simulink model "pfb_fir_256c_2p_16i_8b_core"  (R2019a)
(part 3 of 29)

      mask prompts: mult_latency "Multiplier Latency"; coeff_width "Coefficient Bit Width In"; coeff_frac_width "Coefficient Fractional Bits"; delay "Data/Sync Delay"; data_width "Data Bit Width In"; bram_latency "BRAM Latency"; use_hdl "Use behavioral HDL for multlipliers"; use_embedded "Use embedded multipliers"
      mask init: same as pfb_fir_256c_2p_16i_8b_core/pfb_fir/pol1_in10_tap2
      mask Callback use_hdl:
      | use_hdl = get_param(gcb,'use_hdl');
      | if( strcmp(use_hdl,'on')),
      |     set_param(gcb, 'use_embedded','off');
      |     set_param(gcb, 'MaskVisibilities',{'on','on','on','on','on','on','on','off'});
      | else,
      |     set_param(gcb, 'MaskVisibilities',{'on','on','on','on','on','on','on','on'});
      | end
  pol1_in8_tap7 : Subsystem  AncestorBlock=casper_library_pfbs/tap  mask(tap){mult_latency=2, coeff_width=18, coeff_frac_width=17, delay=16, data_width=8, bram_latency=2, use_hdl=on, use_embedded=off}
      mask prompts: mult_latency "Multiplier Latency"; coeff_width "Coefficient Bit Width In"; coeff_frac_width "Coefficient Fractional Bits"; delay "Data/Sync Delay"; data_width "Data Bit Width In"; bram_latency "BRAM Latency"; use_hdl "Use behavioral HDL for multlipliers"; use_embedded "Use embedded multipliers"
      mask init: same as pfb_fir_256c_2p_16i_8b_core/pfb_fir/pol1_in10_tap2
      mask Callback use_hdl:
      | use_hdl = get_param(gcb,'use_hdl');
      | if( strcmp(use_hdl,'on')),
      |     set_param(gcb, 'use_embedded','off');
      |     set_param(gcb, 'MaskVisibilities',{'on','on','on','on','on','on','on','off'});
      | else,
      |     set_param(gcb, 'MaskVisibilities',{'on','on','on','on','on','on','on','on'});
      | end
  pol1_in9_coeffs : Subsystem  AncestorBlock=casper_library_pfbs/pfb_coeff_gen  mask(pfb_coeff_gen){PFBSize=8, CoeffBitWidth=18, TotalTaps=8, CoeffDistMem=off, WindowType=hamming, bram_latency=2, n_inputs=4, nput=8, fwidth=1, debug_mode=off, fan_latency=1}
      mask prompts: PFBSize "Size of PFB: (2^? pnts)"; CoeffBitWidth "Bitwidth of Coefficients:"; TotalTaps "Total Number of Taps:"; CoeffDistMem "Implement Coeff Gen in Distributed Memory"; WindowType "Windowing Function:"; bram_latency "BRAM Latency"; n_inputs "Number of Simultaneous Inputs: (2^?)"; nput "This is input number:"; fwidth "Bin Width (normal=1)"; debug_mode "Debug mode - coeffs are a [1:pfb_size*taps] ramp."; fan_latency "Fanout latency"
      mask init: same as pfb_fir_256c_2p_16i_8b_core/pfb_fir/pol1_in10_coeffs
      settings: AttributesFormatString=|
      | PFBSize=8, n_inputs=4,
      | taps=8, input=8
  pol1_in9_first_tap : Subsystem  AncestorBlock=casper_library_pfbs/first_tap  mask(first_tap){PFBSize=8, CoeffBitWidth=18, TotalTaps=8, BitWidthIn=8, WindowType=hamming, mult_latency=2, bram_latency=2, n_inputs=4, fwidth=1, use_hdl=on, use_embedded=off}
      mask prompts: PFBSize "Size of PFB: (2^? pnts)"; CoeffBitWidth "Bitwidth of Coefficients:"; TotalTaps "Total Number of Taps:"; BitWidthIn "Input Bitwidth:"; WindowType "Windowing Function:"; mult_latency "Mult Latency"; bram_latency "BRAM Latency"; n_inputs "Number of Simultaneous Inputs: (2^?)"; fwidth "Bit Width (normal=1)"; use_hdl "Use behavioral HDL for multlipliers"; use_embedded "Use embedded multipliers"
      mask init: same as pfb_fir_256c_2p_16i_8b_core/pfb_fir/pol1_in10_first_tap
      settings: AttributesFormatString=taps=8
      mask TypeOptions WindowType: bartlett | barthannwin | blackman | blackmanharris | bohamwin | chebwin | flattopwin | gausswin | hamming | hann | kaiser | nuttallwin | parzenwin | rectwin | tukeywin | triang
      mask Callback use_hdl:
      | use_hdl = get_param(gcb,'use_hdl');
      | if( strcmp(use_hdl,'on')),
      |     set_param(gcb, 'use_embedded','off');
      |     set_param(gcb, 'MaskVisibilities',{'on','on','on','on','on','on','on','on','on','on','off'});
      | else,
      |     set_param(gcb, 'MaskVisibilities',{'on','on','on','on','on','on','on','on','on','on','on'});
      | end
  pol1_in9_last_tap : Subsystem  AncestorBlock=casper_library_pfbs/last_tap  mask(last_tap){TotalTaps=8, BitWidthIn=8, BitWidthOut=18, CoeffBitWidth=18, add_latency=1, mult_latency=2, quantization=Round  (unbiased: Even Values), use_hdl=on, use_embedded=off}
      mask prompts: TotalTaps "Total Number of Taps:"; BitWidthIn "Input Bitwidth:"; BitWidthOut "Output Bitwidth:"; CoeffBitWidth "Coeff Bitwidth:"; add_latency "Add Latency"; mult_latency "Mult Latency"; quantization "Quantization Behavior"; use_hdl "Use behavioral HDL for multlipliers"; use_embedded "Use embedded multipliers"
      mask init: same as pfb_fir_256c_2p_16i_8b_core/pfb_fir/pol1_in10_last_tap
      settings: AttributesFormatString=taps=8
      mask TypeOptions quantization: Truncate | Round  (unbiased: +/- Inf) | Round  (unbiased: Even Values)
      mask Callback use_hdl:
      | use_hdl = get_param(gcb,'use_hdl');
      | if( strcmp(use_hdl,'on')),
      |     set_param(gcb, 'use_embedded','off');
      |     set_param(gcb, 'MaskVisibilities',{'on','on','on','on','on','on','on','on','off'});
      | else,
      |     set_param(gcb, 'MaskVisibilities',{'on','on','on','on','on','on','on','on','on'});
      | end
  pol1_in9_tap2 : Subsystem  AncestorBlock=casper_library_pfbs/tap  mask(tap){mult_latency=2, coeff_width=18, coeff_frac_width=17, delay=16, data_width=8, bram_latency=2, use_hdl=on, use_embedded=off}
      mask prompts: mult_latency "Multiplier Latency"; coeff_width "Coefficient Bit Width In"; coeff_frac_width "Coefficient Fractional Bits"; delay "Data/Sync Delay"; data_width "Data Bit Width In"; bram_latency "BRAM Latency"; use_hdl "Use behavioral HDL for multlipliers"; use_embedded "Use embedded multipliers"
      mask init: same as pfb_fir_256c_2p_16i_8b_core/pfb_fir/pol1_in10_tap2
      mask Callback use_hdl:
      | use_hdl = get_param(gcb,'use_hdl');
      | if( strcmp(use_hdl,'on')),
      |     set_param(gcb, 'use_embedded','off');
      |     set_param(gcb, 'MaskVisibilities',{'on','on','on','on','on','on','on','off'});
      | else,
      |     set_param(gcb, 'MaskVisibilities',{'on','on','on','on','on','on','on','on'});
      | end
  pol1_in9_tap3 : Subsystem  AncestorBlock=casper_library_pfbs/tap  mask(tap){mult_latency=2, coeff_width=18, coeff_frac_width=17, delay=16, data_width=8, bram_latency=2, use_hdl=on, use_embedded=off}
      mask prompts: mult_latency "Multiplier Latency"; coeff_width "Coefficient Bit Width In"; coeff_frac_width "Coefficient Fractional Bits"; delay "Data/Sync Delay"; data_width "Data Bit Width In"; bram_latency "BRAM Latency"; use_hdl "Use behavioral HDL for multlipliers"; use_embedded "Use embedded multipliers"
      mask init: same as pfb_fir_256c_2p_16i_8b_core/pfb_fir/pol1_in10_tap2
      mask Callback use_hdl:
      | use_hdl = get_param(gcb,'use_hdl');
      | if( strcmp(use_hdl,'on')),
      |     set_param(gcb, 'use_embedded','off');
      |     set_param(gcb, 'MaskVisibilities',{'on','on','on','on','on','on','on','off'});
      | else,
      |     set_param(gcb, 'MaskVisibilities',{'on','on','on','on','on','on','on','on'});
      | end
  pol1_in9_tap4 : Subsystem  AncestorBlock=casper_library_pfbs/tap  mask(tap){mult_latency=2, coeff_width=18, coeff_frac_width=17, delay=16, data_width=8, bram_latency=2, use_hdl=on, use_embedded=off}
      mask prompts: mult_latency "Multiplier Latency"; coeff_width "Coefficient Bit Width In"; coeff_frac_width "Coefficient Fractional Bits"; delay "Data/Sync Delay"; data_width "Data Bit Width In"; bram_latency "BRAM Latency"; use_hdl "Use behavioral HDL for multlipliers"; use_embedded "Use embedded multipliers"
      mask init: same as pfb_fir_256c_2p_16i_8b_core/pfb_fir/pol1_in10_tap2
      mask Callback use_hdl:
      | use_hdl = get_param(gcb,'use_hdl');
      | if( strcmp(use_hdl,'on')),
      |     set_param(gcb, 'use_embedded','off');
      |     set_param(gcb, 'MaskVisibilities',{'on','on','on','on','on','on','on','off'});
      | else,
      |     set_param(gcb, 'MaskVisibilities',{'on','on','on','on','on','on','on','on'});
      | end
  pol1_in9_tap5 : Subsystem  AncestorBlock=casper_library_pfbs/tap  mask(tap){mult_latency=2, coeff_width=18, coeff_frac_width=17, delay=16, data_width=8, bram_latency=2, use_hdl=on, use_embedded=off}
      mask prompts: mult_latency "Multiplier Latency"; coeff_width "Coefficient Bit Width In"; coeff_frac_width "Coefficient Fractional Bits"; delay "Data/Sync Delay"; data_width "Data Bit Width In"; bram_latency "BRAM Latency"; use_hdl "Use behavioral HDL for multlipliers"; use_embedded "Use embedded multipliers"
      mask init: same as pfb_fir_256c_2p_16i_8b_core/pfb_fir/pol1_in10_tap2
      mask Callback use_hdl:
      | use_hdl = get_param(gcb,'use_hdl');
      | if( strcmp(use_hdl,'on')),
      |     set_param(gcb, 'use_embedded','off');
      |     set_param(gcb, 'MaskVisibilities',{'on','on','on','on','on','on','on','off'});
      | else,
      |     set_param(gcb, 'MaskVisibilities',{'on','on','on','on','on','on','on','on'});
      | end
  pol1_in9_tap6 : Subsystem  AncestorBlock=casper_library_pfbs/tap  mask(tap){mult_latency=2, coeff_width=18, coeff_frac_width=17, delay=16, data_width=8, bram_latency=2, use_hdl=on, use_embedded=off}
      mask prompts: mult_latency "Multiplier Latency"; coeff_width "Coefficient Bit Width In"; coeff_frac_width "Coefficient Fractional Bits"; delay "Data/Sync Delay"; data_width "Data Bit Width In"; bram_latency "BRAM Latency"; use_hdl "Use behavioral HDL for multlipliers"; use_embedded "Use embedded multipliers"
      mask init: same as pfb_fir_256c_2p_16i_8b_core/pfb_fir/pol1_in10_tap2
      mask Callback use_hdl:
      | use_hdl = get_param(gcb,'use_hdl');
      | if( strcmp(use_hdl,'on')),
      |     set_param(gcb, 'use_embedded','off');
      |     set_param(gcb, 'MaskVisibilities',{'on','on','on','on','on','on','on','off'});
      | else,
      |     set_param(gcb, 'MaskVisibilities',{'on','on','on','on','on','on','on','on'});
      | end
  pol1_in9_tap7 : Subsystem  AncestorBlock=casper_library_pfbs/tap  mask(tap){mult_latency=2, coeff_width=18, coeff_frac_width=17, delay=16, data_width=8, bram_latency=2, use_hdl=on, use_embedded=off}
      mask prompts: mult_latency "Multiplier Latency"; coeff_width "Coefficient Bit Width In"; coeff_frac_width "Coefficient Fractional Bits"; delay "Data/Sync Delay"; data_width "Data Bit Width In"; bram_latency "BRAM Latency"; use_hdl "Use behavioral HDL for multlipliers"; use_embedded "Use embedded multipliers"
      mask init: same as pfb_fir_256c_2p_16i_8b_core/pfb_fir/pol1_in10_tap2
      mask Callback use_hdl:
      | use_hdl = get_param(gcb,'use_hdl');
      | if( strcmp(use_hdl,'on')),
      |     set_param(gcb, 'use_embedded','off');
      |     set_param(gcb, 'MaskVisibilities',{'on','on','on','on','on','on','on','off'});
      | else,
      |     set_param(gcb, 'MaskVisibilities',{'on','on','on','on','on','on','on','on'});
      | end
  sync_out : Outport
  pol1_out1 : Outport  Port=2
  pol1_out2 : Outport  Port=3
  pol1_out3 : Outport  Port=4
  pol1_out4 : Outport  Port=5
  pol1_out5 : Outport  Port=6
  pol1_out6 : Outport  Port=7
  pol1_out7 : Outport  Port=8
  pol1_out8 : Outport  Port=9
  pol1_out9 : Outport  Port=10
  pol1_out10 : Outport  Port=11
  pol1_out11 : Outport  Port=12
  pol1_out12 : Outport  Port=13
  pol1_out13 : Outport  Port=14
  pol1_out14 : Outport  Port=15
  pol1_out15 : Outport  Port=16
  pol1_out16 : Outport  Port=17
  wires:
  pol1_in1/1 -> pol1_in1_coeffs/1(din)
  sync/1 -> pol1_in1_coeffs/2(sync), pol1_in2_coeffs/2(sync), pol1_in3_coeffs/2(sync), pol1_in4_coeffs/2(sync), pol1_in5_coeffs/2(sync), pol1_in6_coeffs/2(sync), pol1_in7_coeffs/2(sync), pol1_in8_coeffs/2(sync), pol1_in9_coeffs/2(sync), pol1_in10_coeffs/2(sync), pol1_in11_coeffs/2(sync), pol1_in12_coeffs/2(sync), pol1_in13_coeffs/2(sync), pol1_in14_coeffs/2(sync), pol1_in15_coeffs/2(sync), pol1_in16_coeffs/2(sync)
  pol1_in1_coeffs/1(dout) -> pol1_in1_first_tap/1(din)
  pol1_in1_coeffs/2(sync_out) -> pol1_in1_first_tap/2(sync), pol1_in2_first_tap/2(sync), pol1_in3_first_tap/2(sync), pol1_in4_first_tap/2(sync), pol1_in5_first_tap/2(sync), pol1_in6_first_tap/2(sync), pol1_in7_first_tap/2(sync), pol1_in8_first_tap/2(sync), pol1_in9_first_tap/2(sync), pol1_in10_first_tap/2(sync), pol1_in11_first_tap/2(sync), pol1_in12_first_tap/2(sync), pol1_in13_first_tap/2(sync), pol1_in14_first_tap/2(sync), pol1_in15_first_tap/2(sync), pol1_in16_first_tap/2(sync)
  pol1_in1_coeffs/3(coeff) -> pol1_in1_first_tap/3(coeffs)
  pol1_in1_first_tap/1(dout) -> pol1_in1_tap2/1(din)
  pol1_in1_first_tap/2(sync_out) -> pol1_in1_tap2/2(sync)
  pol1_in1_first_tap/3(coeff_out) -> pol1_in1_tap2/3(coeff)
  pol1_in1_first_tap/4(taps_out) -> pol1_in1_tap2/4(taps)
  pol1_in1_tap2/1(dout) -> pol1_in1_tap3/1(din)
  pol1_in1_tap2/2(sync_out) -> pol1_in1_tap3/2(sync)
  pol1_in1_tap2/3(coeff_out) -> pol1_in1_tap3/3(coeff)
  pol1_in1_tap2/4(taps_out) -> pol1_in1_tap3/4(taps)
  pol1_in1_tap3/1(dout) -> pol1_in1_tap4/1(din)
  pol1_in1_tap3/2(sync_out) -> pol1_in1_tap4/2(sync)
  pol1_in1_tap3/3(coeff_out) -> pol1_in1_tap4/3(coeff)
  pol1_in1_tap3/4(taps_out) -> pol1_in1_tap4/4(taps)
  pol1_in1_tap4/1(dout) -> pol1_in1_tap5/1(din)
  pol1_in1_tap4/2(sync_out) -> pol1_in1_tap5/2(sync)
  pol1_in1_tap4/3(coeff_out) -> pol1_in1_tap5/3(coeff)
  pol1_in1_tap4/4(taps_out) -> pol1_in1_tap5/4(taps)
  pol1_in1_tap5/1(dout) -> pol1_in1_tap6/1(din)
  pol1_in1_tap5/2(sync_out) -> pol1_in1_tap6/2(sync)
  pol1_in1_tap5/3(coeff_out) -> pol1_in1_tap6/3(coeff)
  pol1_in1_tap5/4(taps_out) -> pol1_in1_tap6/4(taps)
  pol1_in1_tap6/1(dout) -> pol1_in1_tap7/1(din)
  pol1_in1_tap6/2(sync_out) -> pol1_in1_tap7/2(sync)
  pol1_in1_tap6/3(coeff_out) -> pol1_in1_tap7/3(coeff)
  pol1_in1_tap6/4(taps_out) -> pol1_in1_tap7/4(taps)
  pol1_in1_tap7/1(dout) -> pol1_in1_last_tap/1(din)
  pol1_in1_tap7/2(sync_out) -> pol1_in1_last_tap/2(sync)
  pol1_in1_tap7/3(coeff_out) -> pol1_in1_last_tap/3(coeff)
  pol1_in1_tap7/4(taps_out) -> pol1_in1_last_tap/4(taps)
  pol1_in1_last_tap/1(dout) -> pol1_out1/1
  pol1_in1_last_tap/2(sync_out) -> sync_out/1
  pol1_in2/1 -> pol1_in2_coeffs/1(din)
  pol1_in2_coeffs/1(dout) -> pol1_in2_first_tap/1(din)
  pol1_in2_coeffs/3(coeff) -> pol1_in2_first_tap/3(coeffs)
  pol1_in2_first_tap/1(dout) -> pol1_in2_tap2/1(din)
  pol1_in2_first_tap/2(sync_out) -> pol1_in2_tap2/2(sync)
  pol1_in2_first_tap/3(coeff_out) -> pol1_in2_tap2/3(coeff)
  pol1_in2_first_tap/4(taps_out) -> pol1_in2_tap2/4(taps)
  pol1_in2_tap2/1(dout) -> pol1_in2_tap3/1(din)
  pol1_in2_tap2/2(sync_out) -> pol1_in2_tap3/2(sync)
  pol1_in2_tap2/3(coeff_out) -> pol1_in2_tap3/3(coeff)
  pol1_in2_tap2/4(taps_out) -> pol1_in2_tap3/4(taps)
  pol1_in2_tap3/1(dout) -> pol1_in2_tap4/1(din)
  pol1_in2_tap3/2(sync_out) -> pol1_in2_tap4/2(sync)
  pol1_in2_tap3/3(coeff_out) -> pol1_in2_tap4/3(coeff)
  pol1_in2_tap3/4(taps_out) -> pol1_in2_tap4/4(taps)
  pol1_in2_tap4/1(dout) -> pol1_in2_tap5/1(din)
  pol1_in2_tap4/2(sync_out) -> pol1_in2_tap5/2(sync)
  pol1_in2_tap4/3(coeff_out) -> pol1_in2_tap5/3(coeff)
  pol1_in2_tap4/4(taps_out) -> pol1_in2_tap5/4(taps)
  pol1_in2_tap5/1(dout) -> pol1_in2_tap6/1(din)
  pol1_in2_tap5/2(sync_out) -> pol1_in2_tap6/2(sync)
  pol1_in2_tap5/3(coeff_out) -> pol1_in2_tap6/3(coeff)
  pol1_in2_tap5/4(taps_out) -> pol1_in2_tap6/4(taps)
  pol1_in2_tap6/1(dout) -> pol1_in2_tap7/1(din)
  pol1_in2_tap6/2(sync_out) -> pol1_in2_tap7/2(sync)
  pol1_in2_tap6/3(coeff_out) -> pol1_in2_tap7/3(coeff)
  pol1_in2_tap6/4(taps_out) -> pol1_in2_tap7/4(taps)
  pol1_in2_tap7/1(dout) -> pol1_in2_last_tap/1(din)
  pol1_in2_tap7/2(sync_out) -> pol1_in2_last_tap/2(sync)
  pol1_in2_tap7/3(coeff_out) -> pol1_in2_last_tap/3(coeff)
  pol1_in2_tap7/4(taps_out) -> pol1_in2_last_tap/4(taps)
  pol1_in2_last_tap/1(dout) -> pol1_out2/1
  pol1_in3/1 -> pol1_in3_coeffs/1(din)
  pol1_in3_coeffs/1(dout) -> pol1_in3_first_tap/1(din)
  pol1_in3_coeffs/3(coeff) -> pol1_in3_first_tap/3(coeffs)
  pol1_in3_first_tap/1(dout) -> pol1_in3_tap2/1(din)
  pol1_in3_first_tap/2(sync_out) -> pol1_in3_tap2/2(sync)
  pol1_in3_first_tap/3(coeff_out) -> pol1_in3_tap2/3(coeff)
  pol1_in3_first_tap/4(taps_out) -> pol1_in3_tap2/4(taps)
  pol1_in3_tap2/1(dout) -> pol1_in3_tap3/1(din)
  pol1_in3_tap2/2(sync_out) -> pol1_in3_tap3/2(sync)
  pol1_in3_tap2/3(coeff_out) -> pol1_in3_tap3/3(coeff)
  pol1_in3_tap2/4(taps_out) -> pol1_in3_tap3/4(taps)
  pol1_in3_tap3/1(dout) -> pol1_in3_tap4/1(din)
  pol1_in3_tap3/2(sync_out) -> pol1_in3_tap4/2(sync)
  pol1_in3_tap3/3(coeff_out) -> pol1_in3_tap4/3(coeff)
  pol1_in3_tap3/4(taps_out) -> pol1_in3_tap4/4(taps)
  pol1_in3_tap4/1(dout) -> pol1_in3_tap5/1(din)
  pol1_in3_tap4/2(sync_out) -> pol1_in3_tap5/2(sync)
  pol1_in3_tap4/3(coeff_out) -> pol1_in3_tap5/3(coeff)
  pol1_in3_tap4/4(taps_out) -> pol1_in3_tap5/4(taps)
  pol1_in3_tap5/1(dout) -> pol1_in3_tap6/1(din)
  pol1_in3_tap5/2(sync_out) -> pol1_in3_tap6/2(sync)
  pol1_in3_tap5/3(coeff_out) -> pol1_in3_tap6/3(coeff)
  pol1_in3_tap5/4(taps_out) -> pol1_in3_tap6/4(taps)
  pol1_in3_tap6/1(dout) -> pol1_in3_tap7/1(din)
  pol1_in3_tap6/2(sync_out) -> pol1_in3_tap7/2(sync)
  pol1_in3_tap6/3(coeff_out) -> pol1_in3_tap7/3(coeff)
  pol1_in3_tap6/4(taps_out) -> pol1_in3_tap7/4(taps)
  pol1_in3_tap7/1(dout) -> pol1_in3_last_tap/1(din)
  pol1_in3_tap7/2(sync_out) -> pol1_in3_last_tap/2(sync)
  pol1_in3_tap7/3(coeff_out) -> pol1_in3_last_tap/3(coeff)
  pol1_in3_tap7/4(taps_out) -> pol1_in3_last_tap/4(taps)
  pol1_in3_last_tap/1(dout) -> pol1_out3/1
  pol1_in4/1 -> pol1_in4_coeffs/1(din)
  pol1_in4_coeffs/1(dout) -> pol1_in4_first_tap/1(din)
  pol1_in4_coeffs/3(coeff) -> pol1_in4_first_tap/3(coeffs)
  pol1_in4_first_tap/1(dout) -> pol1_in4_tap2/1(din)
  pol1_in4_first_tap/2(sync_out) -> pol1_in4_tap2/2(sync)
  pol1_in4_first_tap/3(coeff_out) -> pol1_in4_tap2/3(coeff)
  pol1_in4_first_tap/4(taps_out) -> pol1_in4_tap2/4(taps)
  pol1_in4_tap2/1(dout) -> pol1_in4_tap3/1(din)
  pol1_in4_tap2/2(sync_out) -> pol1_in4_tap3/2(sync)
  pol1_in4_tap2/3(coeff_out) -> pol1_in4_tap3/3(coeff)
  pol1_in4_tap2/4(taps_out) -> pol1_in4_tap3/4(taps)
  pol1_in4_tap3/1(dout) -> pol1_in4_tap4/1(din)
  pol1_in4_tap3/2(sync_out) -> pol1_in4_tap4/2(sync)
  pol1_in4_tap3/3(coeff_out) -> pol1_in4_tap4/3(coeff)
  pol1_in4_tap3/4(taps_out) -> pol1_in4_tap4/4(taps)
  pol1_in4_tap4/1(dout) -> pol1_in4_tap5/1(din)
  pol1_in4_tap4/2(sync_out) -> pol1_in4_tap5/2(sync)
  pol1_in4_tap4/3(coeff_out) -> pol1_in4_tap5/3(coeff)
  pol1_in4_tap4/4(taps_out) -> pol1_in4_tap5/4(taps)
  pol1_in4_tap5/1(dout) -> pol1_in4_tap6/1(din)
  pol1_in4_tap5/2(sync_out) -> pol1_in4_tap6/2(sync)
  pol1_in4_tap5/3(coeff_out) -> pol1_in4_tap6/3(coeff)
  pol1_in4_tap5/4(taps_out) -> pol1_in4_tap6/4(taps)
  pol1_in4_tap6/1(dout) -> pol1_in4_tap7/1(din)
  pol1_in4_tap6/2(sync_out) -> pol1_in4_tap7/2(sync)
  pol1_in4_tap6/3(coeff_out) -> pol1_in4_tap7/3(coeff)
  pol1_in4_tap6/4(taps_out) -> pol1_in4_tap7/4(taps)
  pol1_in4_tap7/1(dout) -> pol1_in4_last_tap/1(din)
  pol1_in4_tap7/2(sync_out) -> pol1_in4_last_tap/2(sync)
  pol1_in4_tap7/3(coeff_out) -> pol1_in4_last_tap/3(coeff)
  pol1_in4_tap7/4(taps_out) -> pol1_in4_last_tap/4(taps)
  pol1_in4_last_tap/1(dout) -> pol1_out4/1
  pol1_in5/1 -> pol1_in5_coeffs/1(din)
  pol1_in5_coeffs/1(dout) -> pol1_in5_first_tap/1(din)
  pol1_in5_coeffs/3(coeff) -> pol1_in5_first_tap/3(coeffs)
  pol1_in5_first_tap/1(dout) -> pol1_in5_tap2/1(din)
  pol1_in5_first_tap/2(sync_out) -> pol1_in5_tap2/2(sync)
  pol1_in5_first_tap/3(coeff_out) -> pol1_in5_tap2/3(coeff)
  pol1_in5_first_tap/4(taps_out) -> pol1_in5_tap2/4(taps)
  pol1_in5_tap2/1(dout) -> pol1_in5_tap3/1(din)
  pol1_in5_tap2/2(sync_out) -> pol1_in5_tap3/2(sync)
  pol1_in5_tap2/3(coeff_out) -> pol1_in5_tap3/3(coeff)
  pol1_in5_tap2/4(taps_out) -> pol1_in5_tap3/4(taps)
  pol1_in5_tap3/1(dout) -> pol1_in5_tap4/1(din)
  pol1_in5_tap3/2(sync_out) -> pol1_in5_tap4/2(sync)
  pol1_in5_tap3/3(coeff_out) -> pol1_in5_tap4/3(coeff)
  pol1_in5_tap3/4(taps_out) -> pol1_in5_tap4/4(taps)
  pol1_in5_tap4/1(dout) -> pol1_in5_tap5/1(din)
  pol1_in5_tap4/2(sync_out) -> pol1_in5_tap5/2(sync)
  pol1_in5_tap4/3(coeff_out) -> pol1_in5_tap5/3(coeff)
  pol1_in5_tap4/4(taps_out) -> pol1_in5_tap5/4(taps)
  pol1_in5_tap5/1(dout) -> pol1_in5_tap6/1(din)
  pol1_in5_tap5/2(sync_out) -> pol1_in5_tap6/2(sync)
  pol1_in5_tap5/3(coeff_out) -> pol1_in5_tap6/3(coeff)
  pol1_in5_tap5/4(taps_out) -> pol1_in5_tap6/4(taps)
  pol1_in5_tap6/1(dout) -> pol1_in5_tap7/1(din)
  pol1_in5_tap6/2(sync_out) -> pol1_in5_tap7/2(sync)
  pol1_in5_tap6/3(coeff_out) -> pol1_in5_tap7/3(coeff)
  pol1_in5_tap6/4(taps_out) -> pol1_in5_tap7/4(taps)
  pol1_in5_tap7/1(dout) -> pol1_in5_last_tap/1(din)
  pol1_in5_tap7/2(sync_out) -> pol1_in5_last_tap/2(sync)
  pol1_in5_tap7/3(coeff_out) -> pol1_in5_last_tap/3(coeff)
  pol1_in5_tap7/4(taps_out) -> pol1_in5_last_tap/4(taps)
  pol1_in5_last_tap/1(dout) -> pol1_out5/1
  pol1_in6/1 -> pol1_in6_coeffs/1(din)
  pol1_in6_coeffs/1(dout) -> pol1_in6_first_tap/1(din)
  pol1_in6_coeffs/3(coeff) -> pol1_in6_first_tap/3(coeffs)
  pol1_in6_first_tap/1(dout) -> pol1_in6_tap2/1(din)
  pol1_in6_first_tap/2(sync_out) -> pol1_in6_tap2/2(sync)
  pol1_in6_first_tap/3(coeff_out) -> pol1_in6_tap2/3(coeff)
  pol1_in6_first_tap/4(taps_out) -> pol1_in6_tap2/4(taps)
  pol1_in6_tap2/1(dout) -> pol1_in6_tap3/1(din)
  pol1_in6_tap2/2(sync_out) -> pol1_in6_tap3/2(sync)
  pol1_in6_tap2/3(coeff_out) -> pol1_in6_tap3/3(coeff)
  pol1_in6_tap2/4(taps_out) -> pol1_in6_tap3/4(taps)
  pol1_in6_tap3/1(dout) -> pol1_in6_tap4/1(din)
  pol1_in6_tap3/2(sync_out) -> pol1_in6_tap4/2(sync)
  pol1_in6_tap3/3(coeff_out) -> pol1_in6_tap4/3(coeff)
  pol1_in6_tap3/4(taps_out) -> pol1_in6_tap4/4(taps)
  pol1_in6_tap4/1(dout) -> pol1_in6_tap5/1(din)
  pol1_in6_tap4/2(sync_out) -> pol1_in6_tap5/2(sync)
  pol1_in6_tap4/3(coeff_out) -> pol1_in6_tap5/3(coeff)
  pol1_in6_tap4/4(taps_out) -> pol1_in6_tap5/4(taps)
  pol1_in6_tap5/1(dout) -> pol1_in6_tap6/1(din)
  pol1_in6_tap5/2(sync_out) -> pol1_in6_tap6/2(sync)
  pol1_in6_tap5/3(coeff_out) -> pol1_in6_tap6/3(coeff)
  pol1_in6_tap5/4(taps_out) -> pol1_in6_tap6/4(taps)
  pol1_in6_tap6/1(dout) -> pol1_in6_tap7/1(din)
  pol1_in6_tap6/2(sync_out) -> pol1_in6_tap7/2(sync)
  pol1_in6_tap6/3(coeff_out) -> pol1_in6_tap7/3(coeff)
  pol1_in6_tap6/4(taps_out) -> pol1_in6_tap7/4(taps)
  pol1_in6_tap7/1(dout) -> pol1_in6_last_tap/1(din)
  pol1_in6_tap7/2(sync_out) -> pol1_in6_last_tap/2(sync)
  pol1_in6_tap7/3(coeff_out) -> pol1_in6_last_tap/3(coeff)
  pol1_in6_tap7/4(taps_out) -> pol1_in6_last_tap/4(taps)
  pol1_in6_last_tap/1(dout) -> pol1_out6/1
  pol1_in7/1 -> pol1_in7_coeffs/1(din)
  pol1_in7_coeffs/1(dout) -> pol1_in7_first_tap/1(din)
  pol1_in7_coeffs/3(coeff) -> pol1_in7_first_tap/3(coeffs)
  pol1_in7_first_tap/1(dout) -> pol1_in7_tap2/1(din)
  pol1_in7_first_tap/2(sync_out) -> pol1_in7_tap2/2(sync)
  pol1_in7_first_tap/3(coeff_out) -> pol1_in7_tap2/3(coeff)
  pol1_in7_first_tap/4(taps_out) -> pol1_in7_tap2/4(taps)
  pol1_in7_tap2/1(dout) -> pol1_in7_tap3/1(din)
  pol1_in7_tap2/2(sync_out) -> pol1_in7_tap3/2(sync)
  pol1_in7_tap2/3(coeff_out) -> pol1_in7_tap3/3(coeff)
  pol1_in7_tap2/4(taps_out) -> pol1_in7_tap3/4(taps)
  pol1_in7_tap3/1(dout) -> pol1_in7_tap4/1(din)
  pol1_in7_tap3/2(sync_out) -> pol1_in7_tap4/2(sync)
  pol1_in7_tap3/3(coeff_out) -> pol1_in7_tap4/3(coeff)
  pol1_in7_tap3/4(taps_out) -> pol1_in7_tap4/4(taps)
  pol1_in7_tap4/1(dout) -> pol1_in7_tap5/1(din)
  pol1_in7_tap4/2(sync_out) -> pol1_in7_tap5/2(sync)
  pol1_in7_tap4/3(coeff_out) -> pol1_in7_tap5/3(coeff)
  pol1_in7_tap4/4(taps_out) -> pol1_in7_tap5/4(taps)
  pol1_in7_tap5/1(dout) -> pol1_in7_tap6/1(din)
  pol1_in7_tap5/2(sync_out) -> pol1_in7_tap6/2(sync)
  pol1_in7_tap5/3(coeff_out) -> pol1_in7_tap6/3(coeff)
  pol1_in7_tap5/4(taps_out) -> pol1_in7_tap6/4(taps)
  pol1_in7_tap6/1(dout) -> pol1_in7_tap7/1(din)
  pol1_in7_tap6/2(sync_out) -> pol1_in7_tap7/2(sync)
  pol1_in7_tap6/3(coeff_out) -> pol1_in7_tap7/3(coeff)
  pol1_in7_tap6/4(taps_out) -> pol1_in7_tap7/4(taps)
  pol1_in7_tap7/1(dout) -> pol1_in7_last_tap/1(din)
  pol1_in7_tap7/2(sync_out) -> pol1_in7_last_tap/2(sync)
  pol1_in7_tap7/3(coeff_out) -> pol1_in7_last_tap/3(coeff)
  pol1_in7_tap7/4(taps_out) -> pol1_in7_last_tap/4(taps)
  pol1_in7_last_tap/1(dout) -> pol1_out7/1
  pol1_in8/1 -> pol1_in8_coeffs/1(din)
  pol1_in8_coeffs/1(dout) -> pol1_in8_first_tap/1(din)
  pol1_in8_coeffs/3(coeff) -> pol1_in8_first_tap/3(coeffs)
  pol1_in8_first_tap/1(dout) -> pol1_in8_tap2/1(din)
  pol1_in8_first_tap/2(sync_out) -> pol1_in8_tap2/2(sync)
  pol1_in8_first_tap/3(coeff_out) -> pol1_in8_tap2/3(coeff)
  pol1_in8_first_tap/4(taps_out) -> pol1_in8_tap2/4(taps)
  pol1_in8_tap2/1(dout) -> pol1_in8_tap3/1(din)
  pol1_in8_tap2/2(sync_out) -> pol1_in8_tap3/2(sync)
  pol1_in8_tap2/3(coeff_out) -> pol1_in8_tap3/3(coeff)
  pol1_in8_tap2/4(taps_out) -> pol1_in8_tap3/4(taps)
  pol1_in8_tap3/1(dout) -> pol1_in8_tap4/1(din)
  pol1_in8_tap3/2(sync_out) -> pol1_in8_tap4/2(sync)
  pol1_in8_tap3/3(coeff_out) -> pol1_in8_tap4/3(coeff)
  pol1_in8_tap3/4(taps_out) -> pol1_in8_tap4/4(taps)
  pol1_in8_tap4/1(dout) -> pol1_in8_tap5/1(din)
  pol1_in8_tap4/2(sync_out) -> pol1_in8_tap5/2(sync)
  pol1_in8_tap4/3(coeff_out) -> pol1_in8_tap5/3(coeff)
  pol1_in8_tap4/4(taps_out) -> pol1_in8_tap5/4(taps)
  pol1_in8_tap5/1(dout) -> pol1_in8_tap6/1(din)
  pol1_in8_tap5/2(sync_out) -> pol1_in8_tap6/2(sync)
  pol1_in8_tap5/3(coeff_out) -> pol1_in8_tap6/3(coeff)
  pol1_in8_tap5/4(taps_out) -> pol1_in8_tap6/4(taps)
  pol1_in8_tap6/1(dout) -> pol1_in8_tap7/1(din)
  pol1_in8_tap6/2(sync_out) -> pol1_in8_tap7/2(sync)
  pol1_in8_tap6/3(coeff_out) -> pol1_in8_tap7/3(coeff)
  pol1_in8_tap6/4(taps_out) -> pol1_in8_tap7/4(taps)
  pol1_in8_tap7/1(dout) -> pol1_in8_last_tap/1(din)
  pol1_in8_tap7/2(sync_out) -> pol1_in8_last_tap/2(sync)
  pol1_in8_tap7/3(coeff_out) -> pol1_in8_last_tap/3(coeff)
  pol1_in8_tap7/4(taps_out) -> pol1_in8_last_tap/4(taps)
  pol1_in8_last_tap/1(dout) -> pol1_out8/1
  pol1_in9/1 -> pol1_in9_coeffs/1(din)
  pol1_in9_coeffs/1(dout) -> pol1_in9_first_tap/1(din)
  pol1_in9_coeffs/3(coeff) -> pol1_in9_first_tap/3(coeffs)
  pol1_in9_first_tap/1(dout) -> pol1_in9_tap2/1(din)
  pol1_in9_first_tap/2(sync_out) -> pol1_in9_tap2/2(sync)
  pol1_in9_first_tap/3(coeff_out) -> pol1_in9_tap2/3(coeff)
  pol1_in9_first_tap/4(taps_out) -> pol1_in9_tap2/4(taps)
  pol1_in9_tap2/1(dout) -> pol1_in9_tap3/1(din)
  pol1_in9_tap2/2(sync_out) -> pol1_in9_tap3/2(sync)
  pol1_in9_tap2/3(coeff_out) -> pol1_in9_tap3/3(coeff)
  pol1_in9_tap2/4(taps_out) -> pol1_in9_tap3/4(taps)
  pol1_in9_tap3/1(dout) -> pol1_in9_tap4/1(din)
  pol1_in9_tap3/2(sync_out) -> pol1_in9_tap4/2(sync)
  pol1_in9_tap3/3(coeff_out) -> pol1_in9_tap4/3(coeff)
  pol1_in9_tap3/4(taps_out) -> pol1_in9_tap4/4(taps)
  pol1_in9_tap4/1(dout) -> pol1_in9_tap5/1(din)
  pol1_in9_tap4/2(sync_out) -> pol1_in9_tap5/2(sync)
  pol1_in9_tap4/3(coeff_out) -> pol1_in9_tap5/3(coeff)
  pol1_in9_tap4/4(taps_out) -> pol1_in9_tap5/4(taps)
  pol1_in9_tap5/1(dout) -> pol1_in9_tap6/1(din)
  pol1_in9_tap5/2(sync_out) -> pol1_in9_tap6/2(sync)
  pol1_in9_tap5/3(coeff_out) -> pol1_in9_tap6/3(coeff)
  pol1_in9_tap5/4(taps_out) -> pol1_in9_tap6/4(taps)
  pol1_in9_tap6/1(dout) -> pol1_in9_tap7/1(din)
  pol1_in9_tap6/2(sync_out) -> pol1_in9_tap7/2(sync)
  pol1_in9_tap6/3(coeff_out) -> pol1_in9_tap7/3(coeff)
  pol1_in9_tap6/4(taps_out) -> pol1_in9_tap7/4(taps)
  pol1_in9_tap7/1(dout) -> pol1_in9_last_tap/1(din)
  pol1_in9_tap7/2(sync_out) -> pol1_in9_last_tap/2(sync)
  pol1_in9_tap7/3(coeff_out) -> pol1_in9_last_tap/3(coeff)
  pol1_in9_tap7/4(taps_out) -> pol1_in9_last_tap/4(taps)
  pol1_in9_last_tap/1(dout) -> pol1_out9/1
  pol1_in10/1 -> pol1_in10_coeffs/1(din)
  pol1_in10_coeffs/1(dout) -> pol1_in10_first_tap/1(din)
  pol1_in10_coeffs/3(coeff) -> pol1_in10_first_tap/3(coeffs)
  pol1_in10_first_tap/1(dout) -> pol1_in10_tap2/1(din)
  pol1_in10_first_tap/2(sync_out) -> pol1_in10_tap2/2(sync)
  pol1_in10_first_tap/3(coeff_out) -> pol1_in10_tap2/3(coeff)
  pol1_in10_first_tap/4(taps_out) -> pol1_in10_tap2/4(taps)
  pol1_in10_tap2/1(dout) -> pol1_in10_tap3/1(din)
  pol1_in10_tap2/2(sync_out) -> pol1_in10_tap3/2(sync)
  pol1_in10_tap2/3(coeff_out) -> pol1_in10_tap3/3(coeff)
  pol1_in10_tap2/4(taps_out) -> pol1_in10_tap3/4(taps)
  pol1_in10_tap3/1(dout) -> pol1_in10_tap4/1(din)
  pol1_in10_tap3/2(sync_out) -> pol1_in10_tap4/2(sync)
  pol1_in10_tap3/3(coeff_out) -> pol1_in10_tap4/3(coeff)
  pol1_in10_tap3/4(taps_out) -> pol1_in10_tap4/4(taps)
  pol1_in10_tap4/1(dout) -> pol1_in10_tap5/1(din)
  pol1_in10_tap4/2(sync_out) -> pol1_in10_tap5/2(sync)
  pol1_in10_tap4/3(coeff_out) -> pol1_in10_tap5/3(coeff)
  pol1_in10_tap4/4(taps_out) -> pol1_in10_tap5/4(taps)
  pol1_in10_tap5/1(dout) -> pol1_in10_tap6/1(din)
  pol1_in10_tap5/2(sync_out) -> pol1_in10_tap6/2(sync)
  pol1_in10_tap5/3(coeff_out) -> pol1_in10_tap6/3(coeff)
  pol1_in10_tap5/4(taps_out) -> pol1_in10_tap6/4(taps)
  pol1_in10_tap6/1(dout) -> pol1_in10_tap7/1(din)
  pol1_in10_tap6/2(sync_out) -> pol1_in10_tap7/2(sync)
  pol1_in10_tap6/3(coeff_out) -> pol1_in10_tap7/3(coeff)
  pol1_in10_tap6/4(taps_out) -> pol1_in10_tap7/4(taps)
  pol1_in10_tap7/1(dout) -> pol1_in10_last_tap/1(din)
  pol1_in10_tap7/2(sync_out) -> pol1_in10_last_tap/2(sync)
  pol1_in10_tap7/3(coeff_out) -> pol1_in10_last_tap/3(coeff)
  pol1_in10_tap7/4(taps_out) -> pol1_in10_last_tap/4(taps)
  pol1_in10_last_tap/1(dout) -> pol1_out10/1
  pol1_in11/1 -> pol1_in11_coeffs/1(din)
  pol1_in11_coeffs/1(dout) -> pol1_in11_first_tap/1(din)
  pol1_in11_coeffs/3(coeff) -> pol1_in11_first_tap/3(coeffs)
  pol1_in11_first_tap/1(dout) -> pol1_in11_tap2/1(din)
  pol1_in11_first_tap/2(sync_out) -> pol1_in11_tap2/2(sync)
  pol1_in11_first_tap/3(coeff_out) -> pol1_in11_tap2/3(coeff)
  pol1_in11_first_tap/4(taps_out) -> pol1_in11_tap2/4(taps)
  pol1_in11_tap2/1(dout) -> pol1_in11_tap3/1(din)
  pol1_in11_tap2/2(sync_out) -> pol1_in11_tap3/2(sync)
  pol1_in11_tap2/3(coeff_out) -> pol1_in11_tap3/3(coeff)
  pol1_in11_tap2/4(taps_out) -> pol1_in11_tap3/4(taps)
  pol1_in11_tap3/1(dout) -> pol1_in11_tap4/1(din)
  pol1_in11_tap3/2(sync_out) -> pol1_in11_tap4/2(sync)
  pol1_in11_tap3/3(coeff_out) -> pol1_in11_tap4/3(coeff)
  pol1_in11_tap3/4(taps_out) -> pol1_in11_tap4/4(taps)
  pol1_in11_tap4/1(dout) -> pol1_in11_tap5/1(din)
  pol1_in11_tap4/2(sync_out) -> pol1_in11_tap5/2(sync)
  pol1_in11_tap4/3(coeff_out) -> pol1_in11_tap5/3(coeff)
  pol1_in11_tap4/4(taps_out) -> pol1_in11_tap5/4(taps)
  pol1_in11_tap5/1(dout) -> pol1_in11_tap6/1(din)
  pol1_in11_tap5/2(sync_out) -> pol1_in11_tap6/2(sync)
  pol1_in11_tap5/3(coeff_out) -> pol1_in11_tap6/3(coeff)
  pol1_in11_tap5/4(taps_out) -> pol1_in11_tap6/4(taps)
  pol1_in11_tap6/1(dout) -> pol1_in11_tap7/1(din)
  pol1_in11_tap6/2(sync_out) -> pol1_in11_tap7/2(sync)
  pol1_in11_tap6/3(coeff_out) -> pol1_in11_tap7/3(coeff)
  pol1_in11_tap6/4(taps_out) -> pol1_in11_tap7/4(taps)
  pol1_in11_tap7/1(dout) -> pol1_in11_last_tap/1(din)
  pol1_in11_tap7/2(sync_out) -> pol1_in11_last_tap/2(sync)
  pol1_in11_tap7/3(coeff_out) -> pol1_in11_last_tap/3(coeff)
  pol1_in11_tap7/4(taps_out) -> pol1_in11_last_tap/4(taps)
  pol1_in11_last_tap/1(dout) -> pol1_out11/1
  pol1_in12/1 -> pol1_in12_coeffs/1(din)
  pol1_in12_coeffs/1(dout) -> pol1_in12_first_tap/1(din)
  pol1_in12_coeffs/3(coeff) -> pol1_in12_first_tap/3(coeffs)
  pol1_in12_first_tap/1(dout) -> pol1_in12_tap2/1(din)
  pol1_in12_first_tap/2(sync_out) -> pol1_in12_tap2/2(sync)
  pol1_in12_first_tap/3(coeff_out) -> pol1_in12_tap2/3(coeff)
  pol1_in12_first_tap/4(taps_out) -> pol1_in12_tap2/4(taps)
  pol1_in12_tap2/1(dout) -> pol1_in12_tap3/1(din)
  pol1_in12_tap2/2(sync_out) -> pol1_in12_tap3/2(sync)
  pol1_in12_tap2/3(coeff_out) -> pol1_in12_tap3/3(coeff)
  pol1_in12_tap2/4(taps_out) -> pol1_in12_tap3/4(taps)
  pol1_in12_tap3/1(dout) -> pol1_in12_tap4/1(din)
  pol1_in12_tap3/2(sync_out) -> pol1_in12_tap4/2(sync)
  pol1_in12_tap3/3(coeff_out) -> pol1_in12_tap4/3(coeff)
  pol1_in12_tap3/4(taps_out) -> pol1_in12_tap4/4(taps)
  pol1_in12_tap4/1(dout) -> pol1_in12_tap5/1(din)
  pol1_in12_tap4/2(sync_out) -> pol1_in12_tap5/2(sync)
  pol1_in12_tap4/3(coeff_out) -> pol1_in12_tap5/3(coeff)
  pol1_in12_tap4/4(taps_out) -> pol1_in12_tap5/4(taps)
  pol1_in12_tap5/1(dout) -> pol1_in12_tap6/1(din)
  pol1_in12_tap5/2(sync_out) -> pol1_in12_tap6/2(sync)
  pol1_in12_tap5/3(coeff_out) -> pol1_in12_tap6/3(coeff)
  pol1_in12_tap5/4(taps_out) -> pol1_in12_tap6/4(taps)
  pol1_in12_tap6/1(dout) -> pol1_in12_tap7/1(din)
  pol1_in12_tap6/2(sync_out) -> pol1_in12_tap7/2(sync)
  pol1_in12_tap6/3(coeff_out) -> pol1_in12_tap7/3(coeff)
  pol1_in12_tap6/4(taps_out) -> pol1_in12_tap7/4(taps)
  pol1_in12_tap7/1(dout) -> pol1_in12_last_tap/1(din)
  pol1_in12_tap7/2(sync_out) -> pol1_in12_last_tap/2(sync)
  pol1_in12_tap7/3(coeff_out) -> pol1_in12_last_tap/3(coeff)
  pol1_in12_tap7/4(taps_out) -> pol1_in12_last_tap/4(taps)
  pol1_in12_last_tap/1(dout) -> pol1_out12/1
  pol1_in13/1 -> pol1_in13_coeffs/1(din)
  pol1_in13_coeffs/1(dout) -> pol1_in13_first_tap/1(din)
  pol1_in13_coeffs/3(coeff) -> pol1_in13_first_tap/3(coeffs)
  pol1_in13_first_tap/1(dout) -> pol1_in13_tap2/1(din)
  pol1_in13_first_tap/2(sync_out) -> pol1_in13_tap2/2(sync)
  pol1_in13_first_tap/3(coeff_out) -> pol1_in13_tap2/3(coeff)
  pol1_in13_first_tap/4(taps_out) -> pol1_in13_tap2/4(taps)
  pol1_in13_tap2/1(dout) -> pol1_in13_tap3/1(din)
  pol1_in13_tap2/2(sync_out) -> pol1_in13_tap3/2(sync)
  pol1_in13_tap2/3(coeff_out) -> pol1_in13_tap3/3(coeff)
  pol1_in13_tap2/4(taps_out) -> pol1_in13_tap3/4(taps)
  pol1_in13_tap3/1(dout) -> pol1_in13_tap4/1(din)
  pol1_in13_tap3/2(sync_out) -> pol1_in13_tap4/2(sync)
  pol1_in13_tap3/3(coeff_out) -> pol1_in13_tap4/3(coeff)
  pol1_in13_tap3/4(taps_out) -> pol1_in13_tap4/4(taps)
  pol1_in13_tap4/1(dout) -> pol1_in13_tap5/1(din)
  pol1_in13_tap4/2(sync_out) -> pol1_in13_tap5/2(sync)
  pol1_in13_tap4/3(coeff_out) -> pol1_in13_tap5/3(coeff)
  pol1_in13_tap4/4(taps_out) -> pol1_in13_tap5/4(taps)
  pol1_in13_tap5/1(dout) -> pol1_in13_tap6/1(din)
  pol1_in13_tap5/2(sync_out) -> pol1_in13_tap6/2(sync)
  pol1_in13_tap5/3(coeff_out) -> pol1_in13_tap6/3(coeff)
  pol1_in13_tap5/4(taps_out) -> pol1_in13_tap6/4(taps)
  pol1_in13_tap6/1(dout) -> pol1_in13_tap7/1(din)
  pol1_in13_tap6/2(sync_out) -> pol1_in13_tap7/2(sync)
  pol1_in13_tap6/3(coeff_out) -> pol1_in13_tap7/3(coeff)
  pol1_in13_tap6/4(taps_out) -> pol1_in13_tap7/4(taps)
  pol1_in13_tap7/1(dout) -> pol1_in13_last_tap/1(din)
  pol1_in13_tap7/2(sync_out) -> pol1_in13_last_tap/2(sync)
  pol1_in13_tap7/3(coeff_out) -> pol1_in13_last_tap/3(coeff)
  pol1_in13_tap7/4(taps_out) -> pol1_in13_last_tap/4(taps)
  pol1_in13_last_tap/1(dout) -> pol1_out13/1
  pol1_in14/1 -> pol1_in14_coeffs/1(din)
  pol1_in14_coeffs/1(dout) -> pol1_in14_first_tap/1(din)
  pol1_in14_coeffs/3(coeff) -> pol1_in14_first_tap/3(coeffs)
  pol1_in14_first_tap/1(dout) -> pol1_in14_tap2/1(din)
  pol1_in14_first_tap/2(sync_out) -> pol1_in14_tap2/2(sync)
  pol1_in14_first_tap/3(coeff_out) -> pol1_in14_tap2/3(coeff)
  pol1_in14_first_tap/4(taps_out) -> pol1_in14_tap2/4(taps)
  pol1_in14_tap2/1(dout) -> pol1_in14_tap3/1(din)
  pol1_in14_tap2/2(sync_out) -> pol1_in14_tap3/2(sync)
  pol1_in14_tap2/3(coeff_out) -> pol1_in14_tap3/3(coeff)
  pol1_in14_tap2/4(taps_out) -> pol1_in14_tap3/4(taps)
  pol1_in14_tap3/1(dout) -> pol1_in14_tap4/1(din)
  pol1_in14_tap3/2(sync_out) -> pol1_in14_tap4/2(sync)
  pol1_in14_tap3/3(coeff_out) -> pol1_in14_tap4/3(coeff)
  pol1_in14_tap3/4(taps_out) -> pol1_in14_tap4/4(taps)
  pol1_in14_tap4/1(dout) -> pol1_in14_tap5/1(din)
  pol1_in14_tap4/2(sync_out) -> pol1_in14_tap5/2(sync)
  pol1_in14_tap4/3(coeff_out) -> pol1_in14_tap5/3(coeff)
  pol1_in14_tap4/4(taps_out) -> pol1_in14_tap5/4(taps)
  pol1_in14_tap5/1(dout) -> pol1_in14_tap6/1(din)
  pol1_in14_tap5/2(sync_out) -> pol1_in14_tap6/2(sync)
  pol1_in14_tap5/3(coeff_out) -> pol1_in14_tap6/3(coeff)
  pol1_in14_tap5/4(taps_out) -> pol1_in14_tap6/4(taps)
  pol1_in14_tap6/1(dout) -> pol1_in14_tap7/1(din)
  pol1_in14_tap6/2(sync_out) -> pol1_in14_tap7/2(sync)
  pol1_in14_tap6/3(coeff_out) -> pol1_in14_tap7/3(coeff)
  pol1_in14_tap6/4(taps_out) -> pol1_in14_tap7/4(taps)
  pol1_in14_tap7/1(dout) -> pol1_in14_last_tap/1(din)
  pol1_in14_tap7/2(sync_out) -> pol1_in14_last_tap/2(sync)
  pol1_in14_tap7/3(coeff_out) -> pol1_in14_last_tap/3(coeff)
  pol1_in14_tap7/4(taps_out) -> pol1_in14_last_tap/4(taps)
  pol1_in14_last_tap/1(dout) -> pol1_out14/1
  pol1_in15/1 -> pol1_in15_coeffs/1(din)
  pol1_in15_coeffs/1(dout) -> pol1_in15_first_tap/1(din)
  pol1_in15_coeffs/3(coeff) -> pol1_in15_first_tap/3(coeffs)
  pol1_in15_first_tap/1(dout) -> pol1_in15_tap2/1(din)
  pol1_in15_first_tap/2(sync_out) -> pol1_in15_tap2/2(sync)
  pol1_in15_first_tap/3(coeff_out) -> pol1_in15_tap2/3(coeff)
  pol1_in15_first_tap/4(taps_out) -> pol1_in15_tap2/4(taps)
  pol1_in15_tap2/1(dout) -> pol1_in15_tap3/1(din)
  pol1_in15_tap2/2(sync_out) -> pol1_in15_tap3/2(sync)
  pol1_in15_tap2/3(coeff_out) -> pol1_in15_tap3/3(coeff)
  pol1_in15_tap2/4(taps_out) -> pol1_in15_tap3/4(taps)
  pol1_in15_tap3/1(dout) -> pol1_in15_tap4/1(din)
  pol1_in15_tap3/2(sync_out) -> pol1_in15_tap4/2(sync)
  pol1_in15_tap3/3(coeff_out) -> pol1_in15_tap4/3(coeff)
  pol1_in15_tap3/4(taps_out) -> pol1_in15_tap4/4(taps)
  pol1_in15_tap4/1(dout) -> pol1_in15_tap5/1(din)
  pol1_in15_tap4/2(sync_out) -> pol1_in15_tap5/2(sync)
  pol1_in15_tap4/3(coeff_out) -> pol1_in15_tap5/3(coeff)
  pol1_in15_tap4/4(taps_out) -> pol1_in15_tap5/4(taps)
  pol1_in15_tap5/1(dout) -> pol1_in15_tap6/1(din)
  pol1_in15_tap5/2(sync_out) -> pol1_in15_tap6/2(sync)
  pol1_in15_tap5/3(coeff_out) -> pol1_in15_tap6/3(coeff)
  pol1_in15_tap5/4(taps_out) -> pol1_in15_tap6/4(taps)
  pol1_in15_tap6/1(dout) -> pol1_in15_tap7/1(din)
  pol1_in15_tap6/2(sync_out) -> pol1_in15_tap7/2(sync)
  pol1_in15_tap6/3(coeff_out) -> pol1_in15_tap7/3(coeff)
  pol1_in15_tap6/4(taps_out) -> pol1_in15_tap7/4(taps)
  pol1_in15_tap7/1(dout) -> pol1_in15_last_tap/1(din)
  pol1_in15_tap7/2(sync_out) -> pol1_in15_last_tap/2(sync)
  pol1_in15_tap7/3(coeff_out) -> pol1_in15_last_tap/3(coeff)
  pol1_in15_tap7/4(taps_out) -> pol1_in15_last_tap/4(taps)
  pol1_in15_last_tap/1(dout) -> pol1_out15/1
  pol1_in16/1 -> pol1_in16_coeffs/1(din)
  pol1_in16_coeffs/1(dout) -> pol1_in16_first_tap/1(din)
  pol1_in16_coeffs/3(coeff) -> pol1_in16_first_tap/3(coeffs)
  pol1_in16_first_tap/1(dout) -> pol1_in16_tap2/1(din)
  pol1_in16_first_tap/2(sync_out) -> pol1_in16_tap2/2(sync)
  pol1_in16_first_tap/3(coeff_out) -> pol1_in16_tap2/3(coeff)
  pol1_in16_first_tap/4(taps_out) -> pol1_in16_tap2/4(taps)
  pol1_in16_tap2/1(dout) -> pol1_in16_tap3/1(din)
  pol1_in16_tap2/2(sync_out) -> pol1_in16_tap3/2(sync)
  pol1_in16_tap2/3(coeff_out) -> pol1_in16_tap3/3(coeff)
  pol1_in16_tap2/4(taps_out) -> pol1_in16_tap3/4(taps)
  pol1_in16_tap3/1(dout) -> pol1_in16_tap4/1(din)
  pol1_in16_tap3/2(sync_out) -> pol1_in16_tap4/2(sync)
  pol1_in16_tap3/3(coeff_out) -> pol1_in16_tap4/3(coeff)
  pol1_in16_tap3/4(taps_out) -> pol1_in16_tap4/4(taps)
  pol1_in16_tap4/1(dout) -> pol1_in16_tap5/1(din)
  pol1_in16_tap4/2(sync_out) -> pol1_in16_tap5/2(sync)
  pol1_in16_tap4/3(coeff_out) -> pol1_in16_tap5/3(coeff)
  pol1_in16_tap4/4(taps_out) -> pol1_in16_tap5/4(taps)
  pol1_in16_tap5/1(dout) -> pol1_in16_tap6/1(din)
  pol1_in16_tap5/2(sync_out) -> pol1_in16_tap6/2(sync)
  pol1_in16_tap5/3(coeff_out) -> pol1_in16_tap6/3(coeff)
  pol1_in16_tap5/4(taps_out) -> pol1_in16_tap6/4(taps)
  pol1_in16_tap6/1(dout) -> pol1_in16_tap7/1(din)
  pol1_in16_tap6/2(sync_out) -> pol1_in16_tap7/2(sync)
  pol1_in16_tap6/3(coeff_out) -> pol1_in16_tap7/3(coeff)
  pol1_in16_tap6/4(taps_out) -> pol1_in16_tap7/4(taps)
  pol1_in16_tap7/1(dout) -> pol1_in16_last_tap/1(din)
  pol1_in16_tap7/2(sync_out) -> pol1_in16_last_tap/2(sync)
  pol1_in16_tap7/3(coeff_out) -> pol1_in16_last_tap/3(coeff)
  pol1_in16_tap7/4(taps_out) -> pol1_in16_last_tap/4(taps)
  pol1_in16_last_tap/1(dout) -> pol1_out16/1
